simulink subsystem "InversePendulumOnly"  (R2025a)
settings: Solver=VariableStepAuto  StartTime=0.0  StopTime=10.0  RelTol=1e-3
model mask{m_p=0, m_c=0, l_c=0, g=0, J_p=0}
settings Model: Creator=Глеб  LastModifiedBy=Глеб

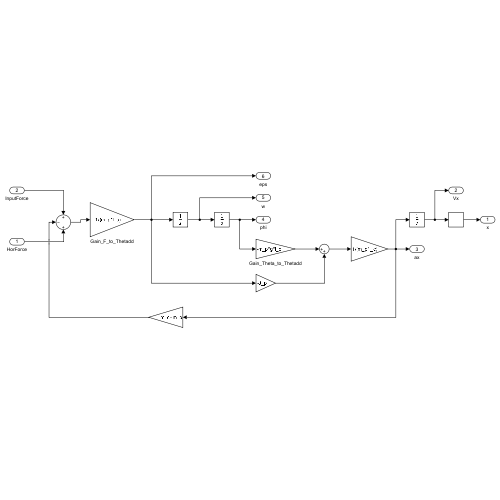
[thumbnail: Simulink's stored preview of the top-level diagram]
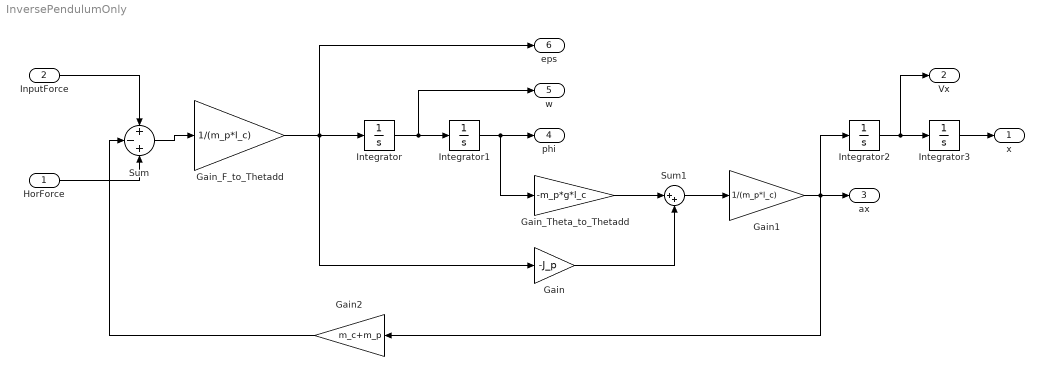
== system InversePendulumOnly ==
  HorForce : Inport
  InputForce : Inport  Port=2
  Gain : Gain  Gain=-J_p
  Gain1 : Gain  Gain=1/(m_p*l_c)
  Gain2 : Gain  Gain=m_c+m_p
  Gain_F_to_Thetadd : Gain  Gain=1/(m_p*l_c)
  Gain_Theta_to_Thetadd : Gain  Gain=-m_p*g*l_c
  Integrator{,1..3} (4 alike) : Integrator
  Sum : Sum  Inputs=+-+
  Sum1 : Sum  Inputs=|++
  x : Outport
  Vx : Outport  Port=2
  ax : Outport  Port=3
  phi : Outport  Port=4
  w : Outport  Port=5
  eps : Outport  Port=6
  wires:
  Sum/1 -> Gain_F_to_Thetadd/1
  InputForce/1 -> Sum/1
  Integrator1/1 -> Gain_Theta_to_Thetadd/1, phi/1
  Gain_Theta_to_Thetadd/1 -> Sum1/1
  Gain_F_to_Thetadd/1 -> eps/1, Integrator/1, Gain/1
  Gain/1 -> Sum1/2
  HorForce/1 -> Sum/3
  Integrator/1 -> w/1, Integrator1/1
  Integrator3/1 -> x/1
  Sum1/1 -> Gain1/1
  Gain2/1 -> Sum/2
  Gain1/1 -> Integrator2/1, Gain2/1, ax/1
  Integrator2/1 -> Vx/1, Integrator3/1
